simulink model "qx"  (R2024b)
settings: Solver=VariableStepAuto  StartTime=0.0  StopTime=10.0  RelTol=1e-3
model workspace (MAT data in the model file):
  Kd = 0
  Ki = 0
  kd = 0
values from neighbouring files (symbols this model uses):
  Kp = 100    [Control_lab2_ex2.m]    (also in Control_lab2_ex3b.m)
settings Model: Creator=googl  LastModifiedBy=googl

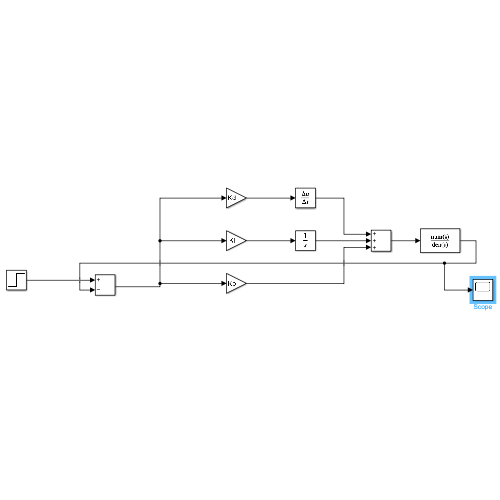
[thumbnail: Simulink's stored preview of the top-level diagram]
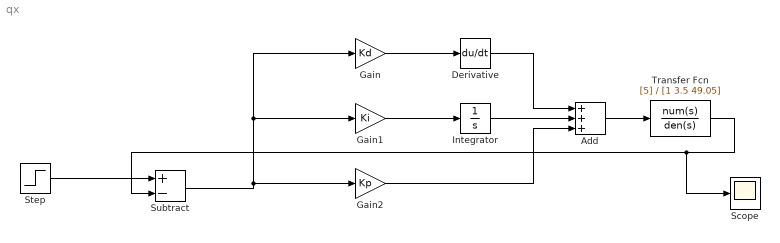
== system qx ==
  Add : Sum  Inputs=+++
  Derivative : Derivative
  Gain : Gain  Gain=Kd
  Gain1 : Gain  Gain=Ki
  Gain2 : Gain  Gain=Kp
  Integrator : Integrator
  Scope : Scope
  Step : Step  SampleTime=0
  Subtract : Sum  Inputs=+-
  Transfer Fcn : TransferFcn  Numerator=[5]  Denominator=[1 3.5 49.05]
  wires:
  Step/1 -> Subtract/1
  Subtract/1 -> Gain/1, Gain1/1, Gain2/1
  Gain/1 -> Derivative/1
  Gain1/1 -> Integrator/1
  Derivative/1 -> Add/1
  Integrator/1 -> Add/2
  Gain2/1 -> Add/3
  Add/1 -> Transfer Fcn/1
  Transfer Fcn/1 -> Scope/1, Subtract/2
